simulink model "LugR7sStEnCtrl"  (R2024b)
settings: Solver=FixedStepDiscrete  StartTime=0.0  StopTime=10.0  FixedStep=0.01  RelTol=1e-3
undefined symbols (not defined in the file or in its folder): data, KeSMSw4SSecRwLtStLgrstOtwdInwdClosePos1_Val, KeSMSw4SSecRwLtStLgrstUpwdDnwdClosePos1_Val, KeSMSw4SSecRwLtStLgrstUpwdDnwdClosePos2_Val, SecRwRtStBkReclnEn_Clear, SecRwRtStBkReclnEn_Set, SecRwRtStFwdBkwdEn_Clear, SecRwRtStFwdBkwdEn_Set, SecRwRtStLgrstInwdOtwdEn_Clear, SecRwRtStLgrstInwdOtwdEn_Set, SecRwRtStLgrstUpwdDnwdEn_Clear, SecRwRtStLgrstUpwdDnwdEn_Set, ThdRwRtStBkReclnEn_Clear, ThdRwRtStBkReclnEn_Set, ThdRwRtStCshnFldEn_Clear, ThdRwRtStCshnFldEn_Set, ThdRwRtStFwdBkwdEn_Clear, ThdRwRtStFwdBkwdEn_Set, ZeroREn_Clear, ZeroREn_Set
libraries: simulink x1
settings Model: Creator=sn2xws  LastModifiedBy=sn55gm
settings Model: ModifiedHistory=|
  | 2024.6.19 V1.0.0 模式流程V1.6
  | 2024.8.2 V3.0.0 模式流程V2.0
  | 2024.8.14 V3.0.1 修复三排前后可能不到位置的问题修复
  | 2024.8.16 V3.0.2腿托和腿托延伸的pos1标定连接错误问题修复
  | 2024.8.23 V3.0.3三右靠背折叠后，未调用前后位置的问题修复
  | 2024.8.26 V3.0.4 模式流程V2.4
  | 2024.9.3 V3.0.5 lug 如果三排折叠已到位，第一阶段会动三排往前的问题
  | 2024.11.15 V3.0.6 md8 md9 同时调用导致2R状态到位被清零，三排前后会重试的问题修复
settings SolverCC: AlgebraicLoopSolver=TrustRegion
settings DataIOCC: SaveFormat=StructureWithTime  ReturnWorkspaceOutputs=off
settings OptimizationCC: DefaultParameterBehavior=Inlined  EnhancedBackFolding=on  PassReuseOutputArgsAs=Individual arguments  ZeroExternalMemoryAtStartup=off  ZeroInternalMemoryAtStartup=off  OptimizeBlockOrder=speed  DifferentSizesBufferReuse=on  OptimizationCustomize=off  EfficientTunableParamExpr=on
settings DebuggingCC: ParameterTunabilityLossMsg=error  UnconnectedInputMsg=warning  UnconnectedOutputMsg=warning  UnconnectedLineMsg=warning  ArithmeticOperatorsInVariantConditions=warning
settings ModelReferenceCC: EnableRefExpFcnMdlSchedulingChecks=on
settings SFSimCC: MATLABDynamicMemAlloc=off  CustomCodeUndefinedFunction=UseInterfaceOnly
settings RTWCC: Description=AUTOSAR  SystemTargetFile=autosar.tlc  GenCodeOnly=on  TemplateMakefile=ert_default_tmf  GenerateReport=on  IncludeHyperlinkInReport=on  LaunchReport=on  DataTypeReplacement=CDataTypesFixedWidth  GenerateTraceInfo=on  GenerateTraceReport=on  GenerateTraceReportSl=on  GenerateTraceReportSf=on  GenerateTraceReportEml=on  GPUComputeCapability=3.5
settings CodeAppCC: ForceParamTrailComments=on  IgnoreCustomStorageClasses=off  OperatorAnnotations=on  SimulinkDataObjDesc=on  SFDataObjDesc=on  InsertBlockDesc=on
settings STFCustomTargetCC: TargetLangStandard=C99 (ISO)  MultiwordLength=256  ParMdlRefBuildCompliant=on  CompOptLevelCompliant=on  IncludeMdlTerminateFcn=off  CombineOutputUpdateFcns=on  SuppressErrorStatus=on  ERTCustomFileBanners=on  SupportNonFinite=off  SupportComplex=off  SupportContinuousTime=off  SupportNonInlinedSFcns=off  RemoveResetFunc=on  MATLABClassNameForMDSCustomization=Simulink.SoftwareTarget.ERTCustomization  AutosarCompliant=on  UseToolchainInfoCompliant=on  LookupTableObjectStructAxisOrder=2,1,3,4,...  LUTObjectStructOrderEvenSpacing=Size,Table,Breakpoints  SystemTargetFile=autosar.tlc
settings ERTTargetCC: TargetLangStandard=C99 (ISO)  ConcurrentExecutionCompliant=off  IncludeMdlTerminateFcn=off  SuppressErrorStatus=on  SupportNonFinite=off  SupportComplex=off  ModelStepFunctionPrototypeControlCompliant=off  CPPClassGenCompliant=off  AutosarCompliant=on  LookupTableObjectStructAxisOrder=2,1,3,4,...  LUTObjectStructOrderEvenSpacing=Size,Table,Breakpoints  ERTCustomFileTemplate=example_file_process.tlc  ERTFilePackagingFormat=Compact  BooleanTrueId=TRUE  BooleanFalseId=FALSE  DynamicArrayContainerType=coder::array

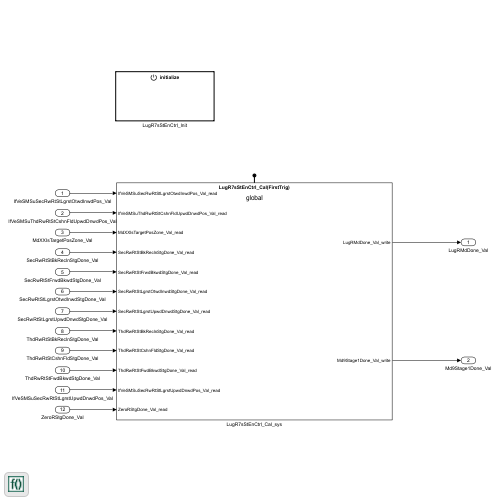
[thumbnail: Simulink's stored preview of the top-level diagram]
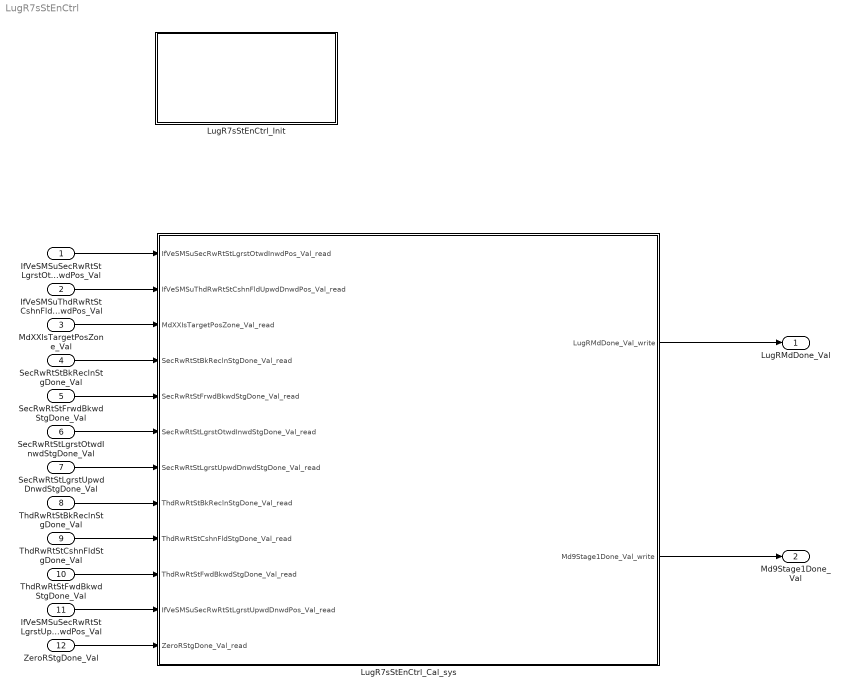
== system LugR7sStEnCtrl ==
  IfVeSMSuSecRwRtStLgrstOtwdInwdPos_Val : Inport  OutDataTypeStr=uint16  PortDimensions=1
  IfVeSMSuThdRwRtStCshnFldUpwdDnwdPos_Val : Inport  Port=2  OutDataTypeStr=uint16  PortDimensions=1
  MdXXIsTargetPosZone_Val : Inport  Port=3  OutDataTypeStr=uint32  PortDimensions=1
  SecRwRtStBkReclnStgDone_Val : Inport  Port=4  OutDataTypeStr=boolean  PortDimensions=1
  SecRwRtStFrwdBkwdStgDone_Val : Inport  Port=5  OutDataTypeStr=boolean  PortDimensions=1
  SecRwRtStLgrstOtwdInwdStgDone_Val : Inport  Port=6  OutDataTypeStr=boolean  PortDimensions=1
  SecRwRtStLgrstUpwdDnwdStgDone_Val : Inport  Port=7  OutDataTypeStr=boolean  PortDimensions=1
  ThdRwRtStBkReclnStgDone_Val : Inport  Port=8  OutDataTypeStr=boolean  PortDimensions=1
  ThdRwRtStCshnFldStgDone_Val : Inport  Port=9  OutDataTypeStr=boolean  PortDimensions=1
  ThdRwRtStFwdBkwdStgDone_Val : Inport  Port=10  OutDataTypeStr=boolean  PortDimensions=1
  IfVeSMSuSecRwRtStLgrstUpwdDnwdPos_Val : Inport  Port=11  OutDataTypeStr=uint16  PortDimensions=1
  ZeroRStgDone_Val : Inport  Port=12  OutDataTypeStr=boolean  PortDimensions=1
  LugR7sStEnCtrl_Cal_sys : Subsystem
  LugR7sStEnCtrl_Init : Subsystem
  LugRMdDone_Val : Outport  OutDataTypeStr=uint8  PortDimensions=1  VectorParamsAs1DForOutWhenUnconnected=off
  Md9Stage1Done_Val : Outport  Port=2  OutDataTypeStr=boolean  PortDimensions=1  VectorParamsAs1DForOutWhenUnconnected=off
  wires:
  IfVeSMSuSecRwRtStLgrstOtwdInwdPos_Val/1 -> LugR7sStEnCtrl_Cal_sys/1(IfVeSMSuSecRwRtStLgrstOtwdInwdPos_Val_read)
  IfVeSMSuThdRwRtStCshnFldUpwdDnwdPos_Val/1 -> LugR7sStEnCtrl_Cal_sys/2(IfVeSMSuThdRwRtStCshnFldUpwdDnwdPos_Val_read)
  MdXXIsTargetPosZone_Val/1 -> LugR7sStEnCtrl_Cal_sys/3(MdXXIsTargetPosZone_Val_read)
  SecRwRtStBkReclnStgDone_Val/1 -> LugR7sStEnCtrl_Cal_sys/4(SecRwRtStBkReclnStgDone_Val_read)
  SecRwRtStFrwdBkwdStgDone_Val/1 -> LugR7sStEnCtrl_Cal_sys/5(SecRwRtStFrwdBkwdStgDone_Val_read)
  SecRwRtStLgrstOtwdInwdStgDone_Val/1 -> LugR7sStEnCtrl_Cal_sys/6(SecRwRtStLgrstOtwdInwdStgDone_Val_read)
  SecRwRtStLgrstUpwdDnwdStgDone_Val/1 -> LugR7sStEnCtrl_Cal_sys/7(SecRwRtStLgrstUpwdDnwdStgDone_Val_read)
  ThdRwRtStBkReclnStgDone_Val/1 -> LugR7sStEnCtrl_Cal_sys/8(ThdRwRtStBkReclnStgDone_Val_read)
  ThdRwRtStCshnFldStgDone_Val/1 -> LugR7sStEnCtrl_Cal_sys/9(ThdRwRtStCshnFldStgDone_Val_read)
  ThdRwRtStFwdBkwdStgDone_Val/1 -> LugR7sStEnCtrl_Cal_sys/10(ThdRwRtStFwdBkwdStgDone_Val_read)
  LugR7sStEnCtrl_Cal_sys/1(LugRMdDone_Val_write) -> LugRMdDone_Val/1
  IfVeSMSuSecRwRtStLgrstUpwdDnwdPos_Val/1 -> LugR7sStEnCtrl_Cal_sys/11(IfVeSMSuSecRwRtStLgrstUpwdDnwdPos_Val_read)
  ZeroRStgDone_Val/1 -> LugR7sStEnCtrl_Cal_sys/12(ZeroRStgDone_Val_read)
  LugR7sStEnCtrl_Cal_sys/2(Md9Stage1Done_Val_write) -> Md9Stage1Done_Val/1

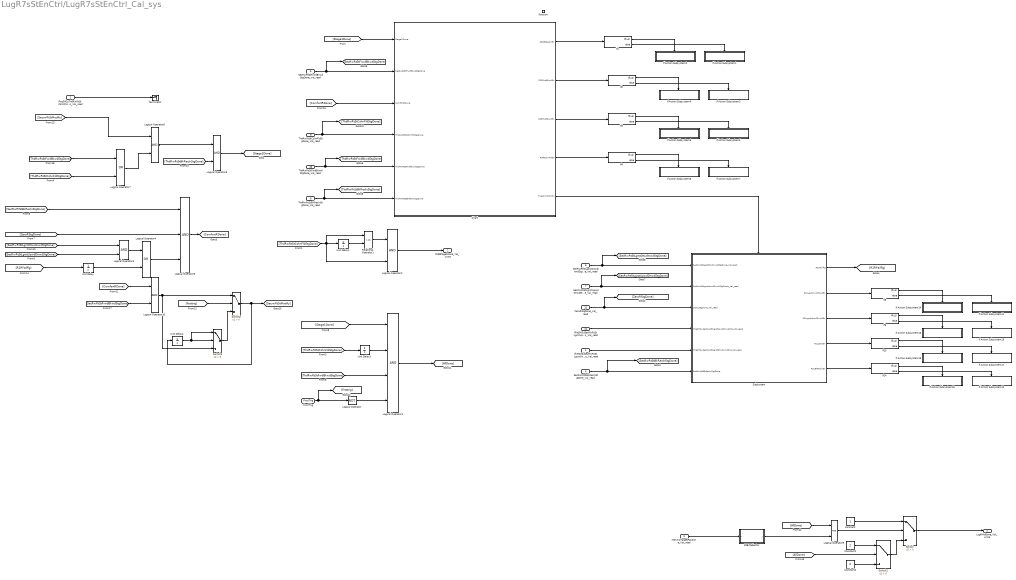
== system LugR7sStEnCtrl/LugR7sStEnCtrl_Cal_sys ==
  IfVeSMSuSecRwRtStLgrstOtwdInwdPos_Val_read : Inport
  IfVeSMSuThdRwRtStCshnFldUpwdDnwdPos_Val_read : Inport  Port=2
  MdXXIsTargetPosZone_Val_read : Inport  Port=3
  SecRwRtStBkReclnStgDone_Val_read : Inport  Port=4
  SecRwRtStFrwdBkwdStgDone_Val_read : Inport  Port=5
  SecRwRtStLgrstOtwdInwdStgDone_Val_read : Inport  Port=6
  SecRwRtStLgrstUpwdDnwdStgDone_Val_read : Inport  Port=7
  ThdRwRtStBkReclnStgDone_Val_read : Inport  Port=8
  ThdRwRtStCshnFldStgDone_Val_read : Inport  Port=9
  ThdRwRtStFwdBkwdStgDone_Val_read : Inport  Port=10
  IfVeSMSuSecRwRtStLgrstUpwdDnwdPos_Val_read : Inport  Port=11
  ZeroRStgDone_Val_read : Inport  Port=12
  function : TriggerPort  TriggerType=function-call  IsSimulinkFunction=on  FunctionName=LugR7sStEnCtrl_Cal  VariantControl=(inherit)
  32BitSelector : Subsystem  mask(32 Bit Selector){BitNum=8}
      mask prompts: BitNum "Select Bit Number"
      mask help: Allows selection of a particular bit (0-31) out of a packed word up to 32 bits long. Output will be true if the bit number selected via the mask parameter is equal to one.
      mask TypeOptions BitNum: 0 | 1 | 2 | 3 | 4 | 5 | 6 | 7 | 8 | 9 | 10 | 11 | 12 | 13 | 14 | 15 | 16 | 17 | 18 | 19 | 20 | 21 | 22 | 23 | 24 | 25 | 26 | 27 | 28 | 29 | 30 | 31
      mask Display:
      | text(0.5, 0.8,'BIT','horizontalAlignment','center')
      | text(0.5, 0.5,'SELECTOR','horizontalAlignment','center')
      | text(0.5, 0.2,['-- Bit ',char(get_param(gcb,'BitNum')),' --'],'horizontalAlignment','center')
  Chart : Stateflow chart  TreatAsAtomicUnit=on
  Constant : Constant  OutDataTypeStr=uint8
  Constant1 : Constant  Value=2  OutDataTypeStr=uint8
  Constant2 : Constant  Value=0  OutDataTypeStr=uint8
  If Action Subsystem1 : Subsystem  TreatAsAtomicUnit=on
  If Action Subsystem11 : Subsystem  TreatAsAtomicUnit=on
  If Action Subsystem12 : Subsystem  TreatAsAtomicUnit=on
  If Action Subsystem14 : Subsystem  TreatAsAtomicUnit=on
  If Action Subsystem15 : Subsystem  TreatAsAtomicUnit=on
  If Action Subsystem16 : Subsystem  TreatAsAtomicUnit=on
  If Action Subsystem17 : Subsystem  TreatAsAtomicUnit=on
  If Action Subsystem18 : Subsystem  TreatAsAtomicUnit=on
  If Action Subsystem2 : Subsystem  TreatAsAtomicUnit=on
  If Action Subsystem25 : Subsystem  TreatAsAtomicUnit=on
  If Action Subsystem3 : Subsystem  TreatAsAtomicUnit=on
  If Action Subsystem4 : Subsystem  TreatAsAtomicUnit=on
  If Action Subsystem5 : Subsystem  TreatAsAtomicUnit=on
  If Action Subsystem6 : Subsystem  TreatAsAtomicUnit=on
  If Action Subsystem7 : Subsystem  TreatAsAtomicUnit=on
  If Action Subsystem8 : Subsystem  TreatAsAtomicUnit=on
  If{1..4,8..10,14} (8 alike) : If  IfExpression=u1
  Logical Operator : Logic  Operator=NOT  AllPortsSameDT=off  OutDataTypeStr=boolean
  Logical Operator1 : Logic  Inputs=4  AllPortsSameDT=off  OutDataTypeStr=boolean
  Logical Operator{2..3,6,8..10} (6 alike) : Logic  AllPortsSameDT=off  OutDataTypeStr=boolean
  Logical Operator4 : Logic  Operator=OR  AllPortsSameDT=off  OutDataTypeStr=boolean
  Logical Operator5 : Logic  Inputs=3  AllPortsSameDT=off  OutDataTypeStr=boolean
  Logical Operator7 : Logic  Operator=OR  AllPortsSameDT=off  OutDataTypeStr=boolean
  Relational Operator1 : RelationalOperator  Operator=~=  OutDataTypeStr=boolean  RndMeth=Simplest  InputSameDT=off
  Subsystem : Subsystem
  Switch{,1..3} (4 alike) : Switch  Criteria=u2 > Threshold  SaturateOnIntegerOverflow=off  InputSameDT=off
  Terminator : Terminator
  Unit Delay{,1..3} (4 alike) : UnitDelay  SampleTime=-1  HasFrameUpgradeWarning=on
  FirstTrig : ArgIn  OutDataTypeStr=boolean  ArgumentName=FirstTrig
  LugRMdDone_Val_write : Outport  VectorParamsAs1DForOutWhenUnconnected=off
      settings: EnsureOutportIsVirtual=on
  Md9Stage1Done_Val_write : Outport  Port=2  VectorParamsAs1DForOutWhenUnconnected=off
      settings: EnsureOutportIsVirtual=on
  wires:
  SecRwRtStBkReclnStgDone_Val_read/1 -> [SecRwRtStBkReclnStgDone], Subsystem/6(SecRwLtStBkReclnStgDone)
  ThdRwRtStCshnFldStgDone_Val_read/1 -> [ThdRwRtStCshnFldStgDone], Chart/4(ThdRwRtStCshnFldStgDone)
  ThdRwRtStFwdBkwdStgDone_Val_read/1 -> [ThdRwRtStFwdBkwdStgDone], Chart/5(ThdRwRtStFwdBkwdStgDone)
  Chart/5(TrigComfortMd()) -> Subsystem/Trigger
  If8/2 -> If Action Subsystem11/Action
  SecRwRtStLgrstOtwdInwdStgDone_Val_read/1 -> [SecRwRtStLgrstOtwdInwdStgDone], Subsystem/1(SecRwLtStLgrstOtwdInwdStgDone_Val_read)
  If14/2 -> If Action Subsystem12/Action
  IfVeSMSuSecRwRtStLgrstOtwdInwdPos_Val_read/1 -> Subsystem/5(IfVeSMSuSecRwLtStLgrstOtwdInwdPos_Val_read)
  Subsystem/3(R2LLgrstUpwdDnwdEn) -> If9/1
  If9/1 -> If Action Subsystem16/Action
  If8/1 -> If Action Subsystem14/Action
  Subsystem/5(R2LBkReclnEn) -> If14/1
  If14/1 -> If Action Subsystem25/Action
  Subsystem/4(R2LZeroEn) -> If10/1
  If10/2 -> If Action Subsystem17/Action
  If9/2 -> If Action Subsystem15/Action
  Subsystem/2(R2LLgrstInwdOtwdEn) -> If8/1
  If10/1 -> If Action Subsystem18/Action
  SecRwRtStLgrstUpwdDnwdStgDone_Val_read/1 -> [SecRwRtStLgrstUpwdDnwdStgDone], Subsystem/2(SecRwLtStLgrstUpwdDnwdStgDone_Val_read)
  Subsystem/1(R2LFailflg) -> [R2RFailflg]
  IfVeSMSuSecRwRtStLgrstUpwdDnwdPos_Val_read/1 -> Subsystem/4(IfVeSMSuSecRwLtStLgrstUpwdDnwdPos_Val_read)
  SecRwRtStFrwdBkwdStgDone_Val_read/1 -> [SecRwRtStFrwdBkwdStgDone], Chart/2(SecRwRtStFrwdBkwdStgDone)
  ThdRwRtStBkReclnStgDone_Val_read/1 -> [ThdRwRtStBkReclnStgDone], Chart/6(ThdRwRtStBkReclnStgDone)
  Logical Operator8/1 -> Logical Operator6/1
  IfVeSMSuThdRwRtStCshnFldUpwdDnwdPos_Val_read/1 -> Terminator/1
  [Stage1Done] -> Chart/1(Stage1Done)
  Unit Delay/1 -> Logical Operator4/2
  Logical Operator5/1 -> [ComfortRDone]
  [SecRwRtStBkReclnStgDone] -> Logical Operator5/1
  [SecRwRtStLgrstUpwdDnwdStgDone] -> Logical Operator3/2
  [R2RFailflg] -> Unit Delay/1
  [ZeroRStgDone] -> Logical Operator5/2
  [SecRwRtStLgrstOtwdInwdStgDone] -> Logical Operator3/1
  Logical Operator4/1 -> Logical Operator5/3
  Logical Operator3/1 -> Logical Operator4/1
  [ComfortRDone] -> Chart/3(ComfortRDone)
  Constant1/1 -> Switch1/1
  MdXXIsTargetPosZone_Val_read/1 -> 32BitSelector/1(x)
  32BitSelector/1(y) -> Logical Operator9/2
  Logical Operator9/1 -> Switch/2
  Switch1/1 -> Switch/3
  Constant2/1 -> Switch1/3
  Switch/1 -> LugRMdDone_Val_write/1
  Constant/1 -> Switch/1
  [AllDone] -> Switch1/2
  [AllDone] -> Logical Operator9/1
  Logical Operator1/1 -> [AllDone]
  [Stage1Done] -> Logical Operator1/1
  ZeroRStgDone_Val_read/1 -> [ZeroRStgDone], Subsystem/3(ZeroLStgDone_Val_read)
  If1/1 -> If Action Subsystem2/Action
  If1/2 -> If Action Subsystem1/Action
  Chart/1(R3RBkReclnEn) -> If1/1
  Chart/2(R2RFwdBkwdEn) -> If2/1
  If2/2 -> If Action Subsystem3/Action
  If2/1 -> If Action Subsystem4/Action
  If3/1 -> If Action Subsystem6/Action
  If3/2 -> If Action Subsystem5/Action
  Chart/3(R3RFwdBkwdEn) -> If3/1
  Chart/4(R3RCshnFldEn) -> If4/1
  If4/2 -> If Action Subsystem7/Action
  If4/1 -> If Action Subsystem8/Action
  Unit Delay1/1 -> Relational Operator1/2
  Logical Operator2/1 -> Md9Stage1Done_Val_write/1
  Relational Operator1/1 -> Logical Operator2/1
  [ThdRwRtStCshnFldStgDone] -> Relational Operator1/1, Logical Operator2/2, Unit Delay1/1
  Logical Operator6/1 -> [Stage1Done]
  [ThdRwRtStBkReclnStgDone] -> Logical Operator6/2
  Unit Delay3/1 -> Logical Operator1/2
  FirstTrig/1 -> [firsttrig], Logical Operator/1
  Logical Operator/1 -> Logical Operator1/4
  Logical Operator7/1 -> Logical Operator8/2
  [ThdRwRtStFwdBkwdStgDone] -> Logical Operator7/1
  [ThdRwRtStCshnFldStgDone] -> Logical Operator7/2
  [ThdRwRtStCshnFldStgDone] -> Unit Delay3/1
  [ThdRwRtStFwdBkwdStgDone] -> Logical Operator1/3
  [firsttrig] -> Switch2/2
  Unit Delay2/1 -> Switch3/1, Switch3/2
  Switch2/1 -> Unit Delay2/1, [SecrwRtStModify]
  Logical Operator10/1 -> Switch3/3, Switch2/1
  Switch3/1 -> Switch2/3
  [ComfortRDone] -> Logical Operator10/1
  [SecRwRtStFrwdBkwdStgDone] -> Logical Operator10/2
  [SecrwRtStModify] -> Logical Operator8/1

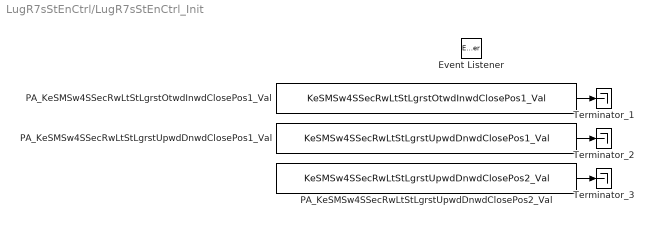
== system LugR7sStEnCtrl/LugR7sStEnCtrl_Init ==
  Event Listener : EventListener  EventName=reset
  PA_KeSMSw4SSecRwLtStLgrstOtwdInwdClosePos1_Val : Constant  Value=KeSMSw4SSecRwLtStLgrstOtwdInwdClosePos1_Val
  PA_KeSMSw4SSecRwLtStLgrstUpwdDnwdClosePos1_Val : Constant  Value=KeSMSw4SSecRwLtStLgrstUpwdDnwdClosePos1_Val
  PA_KeSMSw4SSecRwLtStLgrstUpwdDnwdClosePos2_Val : Constant  Value=KeSMSw4SSecRwLtStLgrstUpwdDnwdClosePos2_Val
  Terminator_1 : Terminator
  Terminator_2 : Terminator
  Terminator_3 : Terminator
  wires:
  PA_KeSMSw4SSecRwLtStLgrstOtwdInwdClosePos1_Val/1 -> Terminator_1/1
  PA_KeSMSw4SSecRwLtStLgrstUpwdDnwdClosePos1_Val/1 -> Terminator_2/1
  PA_KeSMSw4SSecRwLtStLgrstUpwdDnwdClosePos2_Val/1 -> Terminator_3/1

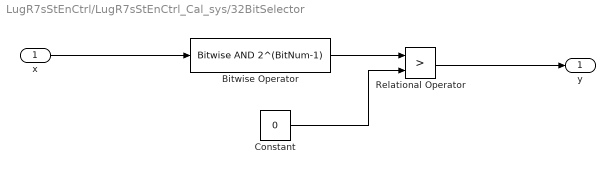
== system LugR7sStEnCtrl/LugR7sStEnCtrl_Cal_sys/32BitSelector ==
  x : Inport
  Bitwise Operator : simulink/Logic and Bit Operations/Bitwise Operator  logicop=AND  UseBitMask=on  BitMask=2^(BitNum-1)  BitMaskRealWorld=Stored Integer
  Constant : Constant  Value=0  OutDataTypeStr=uint32
  Relational Operator : RelationalOperator  Operator=>  OutDataTypeStr=boolean  RndMeth=Simplest  InputSameDT=off
  y : Outport  VectorParamsAs1DForOutWhenUnconnected=off
  wires:
  Relational Operator/1 -> y/1
  Constant/1 -> Relational Operator/2
  x/1 -> Bitwise Operator/1
  Bitwise Operator/1 -> Relational Operator/1

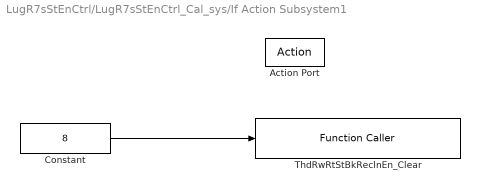
== system LugR7sStEnCtrl/LugR7sStEnCtrl_Cal_sys/If Action Subsystem1 ==
  Action Port : ActionPort  ActionPortLabel=else
  Constant : Constant  Value=8  OutDataTypeStr=uint8
  ThdRwRtStBkReclnEn_Clear : FunctionCaller  FunctionPrototype=ThdRwRtStBkReclnEn_Clear(data)  InputArgumentSpecifications=uint8(1)  OutputArgumentSpecifications=<Enter example>
  wires:
  Constant/1 -> ThdRwRtStBkReclnEn_Clear/1

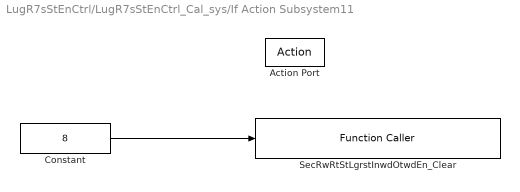
== system LugR7sStEnCtrl/LugR7sStEnCtrl_Cal_sys/If Action Subsystem11 ==
  Action Port : ActionPort  ActionPortLabel=else
  Constant : Constant  Value=8  OutDataTypeStr=uint8
  SecRwRtStLgrstInwdOtwdEn_Clear : FunctionCaller  FunctionPrototype=SecRwRtStLgrstInwdOtwdEn_Clear(data)  InputArgumentSpecifications=uint8(1)  OutputArgumentSpecifications=<Enter example>
  wires:
  Constant/1 -> SecRwRtStLgrstInwdOtwdEn_Clear/1

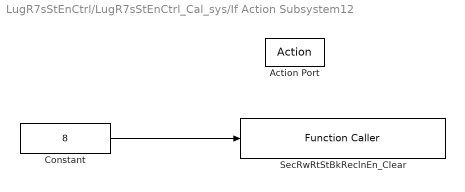
== system LugR7sStEnCtrl/LugR7sStEnCtrl_Cal_sys/If Action Subsystem12 ==
  Action Port : ActionPort  ActionPortLabel=else
  Constant : Constant  Value=8  OutDataTypeStr=uint8
  SecRwRtStBkReclnEn_Clear : FunctionCaller  FunctionPrototype=SecRwRtStBkReclnEn_Clear(data)  InputArgumentSpecifications=uint8(1)  OutputArgumentSpecifications=<Enter example>
  wires:
  Constant/1 -> SecRwRtStBkReclnEn_Clear/1

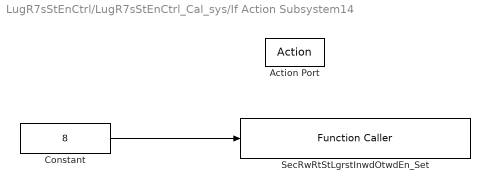
== system LugR7sStEnCtrl/LugR7sStEnCtrl_Cal_sys/If Action Subsystem14 ==
  Action Port : ActionPort  ActionPortLabel=if(u1)
  Constant : Constant  Value=8  OutDataTypeStr=uint8
  SecRwRtStLgrstInwdOtwdEn_Set : FunctionCaller  FunctionPrototype=SecRwRtStLgrstInwdOtwdEn_Set(data)  InputArgumentSpecifications=uint8(1)  OutputArgumentSpecifications=<Enter example>
  wires:
  Constant/1 -> SecRwRtStLgrstInwdOtwdEn_Set/1

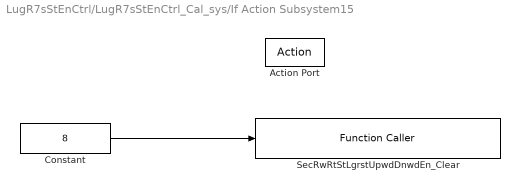
== system LugR7sStEnCtrl/LugR7sStEnCtrl_Cal_sys/If Action Subsystem15 ==
  Action Port : ActionPort  ActionPortLabel=else
  Constant : Constant  Value=8  OutDataTypeStr=uint8
  SecRwRtStLgrstUpwdDnwdEn_Clear : FunctionCaller  FunctionPrototype=SecRwRtStLgrstUpwdDnwdEn_Clear(data)  InputArgumentSpecifications=uint8(1)  OutputArgumentSpecifications=<Enter example>
  wires:
  Constant/1 -> SecRwRtStLgrstUpwdDnwdEn_Clear/1

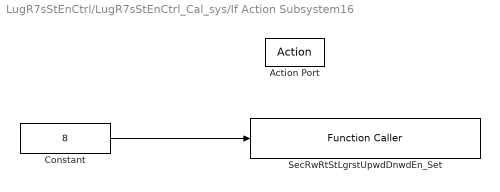
== system LugR7sStEnCtrl/LugR7sStEnCtrl_Cal_sys/If Action Subsystem16 ==
  Action Port : ActionPort  ActionPortLabel=if(u1)
  Constant : Constant  Value=8  OutDataTypeStr=uint8
  SecRwRtStLgrstUpwdDnwdEn_Set : FunctionCaller  FunctionPrototype=SecRwRtStLgrstUpwdDnwdEn_Set(data)  InputArgumentSpecifications=uint8(1)  OutputArgumentSpecifications=<Enter example>
  wires:
  Constant/1 -> SecRwRtStLgrstUpwdDnwdEn_Set/1

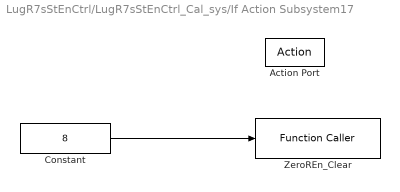
== system LugR7sStEnCtrl/LugR7sStEnCtrl_Cal_sys/If Action Subsystem17 ==
  Action Port : ActionPort  ActionPortLabel=else
  Constant : Constant  Value=8  OutDataTypeStr=uint8
  ZeroREn_Clear : FunctionCaller  FunctionPrototype=ZeroREn_Clear(data)  InputArgumentSpecifications=uint8(1)  OutputArgumentSpecifications=<Enter example>
  wires:
  Constant/1 -> ZeroREn_Clear/1

== system LugR7sStEnCtrl/LugR7sStEnCtrl_Cal_sys/If Action Subsystem18 ==
  Action Port : ActionPort  ActionPortLabel=if(u1)
  Constant : Constant  Value=8  OutDataTypeStr=uint8
  ZeroREn_Set : FunctionCaller  FunctionPrototype=ZeroREn_Set(data)  InputArgumentSpecifications=uint8(1)  OutputArgumentSpecifications=<Enter example>
  wires:
  Constant/1 -> ZeroREn_Set/1

== system LugR7sStEnCtrl/LugR7sStEnCtrl_Cal_sys/If Action Subsystem2 ==
  Action Port : ActionPort  ActionPortLabel=if(u1)
  Constant : Constant  Value=8  OutDataTypeStr=uint8
  ThdRwRtStBkReclnEn_Set : FunctionCaller  FunctionPrototype=ThdRwRtStBkReclnEn_Set(data)  InputArgumentSpecifications=uint8(1)  OutputArgumentSpecifications=<Enter example>
  wires:
  Constant/1 -> ThdRwRtStBkReclnEn_Set/1

== system LugR7sStEnCtrl/LugR7sStEnCtrl_Cal_sys/If Action Subsystem25 ==
  Action Port : ActionPort  ActionPortLabel=if(u1)
  Constant : Constant  Value=8  OutDataTypeStr=uint8
  SecRwRtStBkReclnEn_Set : FunctionCaller  FunctionPrototype=SecRwRtStBkReclnEn_Set(data)  InputArgumentSpecifications=uint8(1)  OutputArgumentSpecifications=<Enter example>
  wires:
  Constant/1 -> SecRwRtStBkReclnEn_Set/1

== system LugR7sStEnCtrl/LugR7sStEnCtrl_Cal_sys/If Action Subsystem3 ==
  Action Port : ActionPort  ActionPortLabel=else
  Constant : Constant  Value=8  OutDataTypeStr=uint8
  SecRwRtStFwdBkwdEn_Clear : FunctionCaller  FunctionPrototype=SecRwRtStFwdBkwdEn_Clear(data)  InputArgumentSpecifications=uint8(1)  OutputArgumentSpecifications=<Enter example>
  wires:
  Constant/1 -> SecRwRtStFwdBkwdEn_Clear/1

== system LugR7sStEnCtrl/LugR7sStEnCtrl_Cal_sys/If Action Subsystem4 ==
  Action Port : ActionPort  ActionPortLabel=if(u1)
  Constant : Constant  Value=8  OutDataTypeStr=uint8
  SecRwRtStFwdBkwdEn_Set : FunctionCaller  FunctionPrototype=SecRwRtStFwdBkwdEn_Set(data)  InputArgumentSpecifications=uint8(1)  OutputArgumentSpecifications=<Enter example>
  wires:
  Constant/1 -> SecRwRtStFwdBkwdEn_Set/1

== system LugR7sStEnCtrl/LugR7sStEnCtrl_Cal_sys/If Action Subsystem5 ==
  Action Port : ActionPort  ActionPortLabel=else
  Constant : Constant  Value=8  OutDataTypeStr=uint8
  ThdRwRtStFwdBkwdEn_Clear : FunctionCaller  FunctionPrototype=ThdRwRtStFwdBkwdEn_Clear(data)  InputArgumentSpecifications=uint8(1)  OutputArgumentSpecifications=<Enter example>
  wires:
  Constant/1 -> ThdRwRtStFwdBkwdEn_Clear/1

== system LugR7sStEnCtrl/LugR7sStEnCtrl_Cal_sys/If Action Subsystem6 ==
  Action Port : ActionPort  ActionPortLabel=if(u1)
  Constant : Constant  Value=8  OutDataTypeStr=uint8
  ThdRwRtStFwdBkwdEn_Set : FunctionCaller  FunctionPrototype=ThdRwRtStFwdBkwdEn_Set(data)  InputArgumentSpecifications=uint8(1)  OutputArgumentSpecifications=<Enter example>
  wires:
  Constant/1 -> ThdRwRtStFwdBkwdEn_Set/1

== system LugR7sStEnCtrl/LugR7sStEnCtrl_Cal_sys/If Action Subsystem7 ==
  Action Port : ActionPort  ActionPortLabel=else
  Constant : Constant  Value=8  OutDataTypeStr=uint8
  ThdRwRtStCshnFldEn_Clear : FunctionCaller  FunctionPrototype=ThdRwRtStCshnFldEn_Clear(data)  InputArgumentSpecifications=uint8(1)  OutputArgumentSpecifications=<Enter example>
  wires:
  Constant/1 -> ThdRwRtStCshnFldEn_Clear/1

== system LugR7sStEnCtrl/LugR7sStEnCtrl_Cal_sys/If Action Subsystem8 ==
  Action Port : ActionPort  ActionPortLabel=if(u1)
  Constant : Constant  Value=8  OutDataTypeStr=uint8
  ThdRwRtStCshnFldEn_Set : FunctionCaller  FunctionPrototype=ThdRwRtStCshnFldEn_Set(data)  InputArgumentSpecifications=uint8(1)  OutputArgumentSpecifications=<Enter example>
  wires:
  Constant/1 -> ThdRwRtStCshnFldEn_Set/1

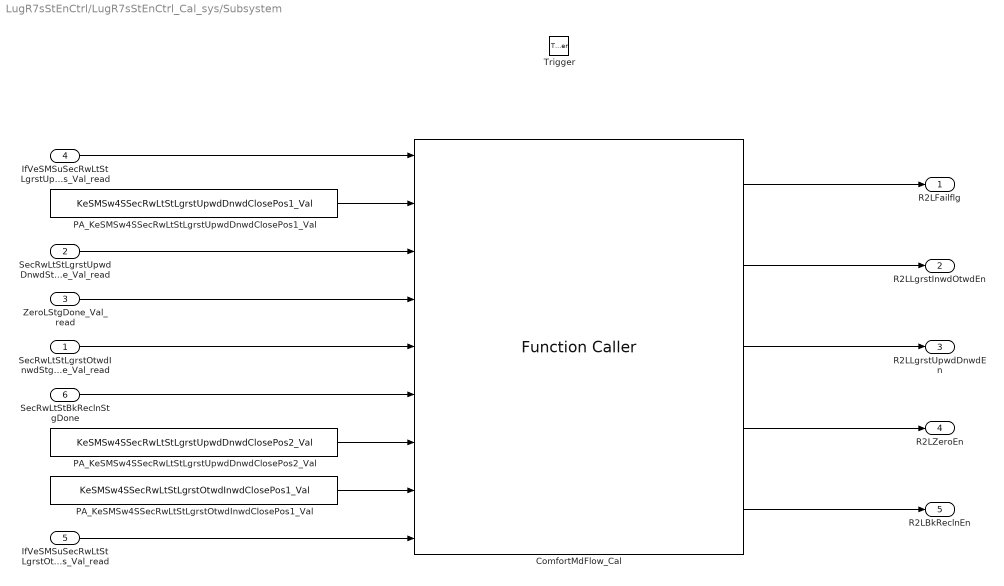
== system LugR7sStEnCtrl/LugR7sStEnCtrl_Cal_sys/Subsystem ==
  SecRwLtStLgrstOtwdInwdStgDone_Val_read : Inport
  SecRwLtStLgrstUpwdDnwdStgDone_Val_read : Inport  Port=2
  ZeroLStgDone_Val_read : Inport  Port=3
  IfVeSMSuSecRwLtStLgrstUpwdDnwdPos_Val_read : Inport  Port=4
  IfVeSMSuSecRwLtStLgrstOtwdInwdPos_Val_read : Inport  Port=5
  SecRwLtStBkReclnStgDone : Inport  Port=6
  Trigger : TriggerPort  TriggerType=function-call  VariantControl=Variant  PortDimensions=1
  ComfortMdFlow_Cal : FunctionCaller  FunctionPrototype=[Failflg,LgrstInwdOtwdEn,LgrstUpwdDnwdEn,ZeroEn,BkReclnEn] = ComfortMdFlow_Cal(LgrstUpwdDnwdPos,LgrstUpwdDnwdClosePos1,LgrstUpwdStgDone,ZeroStgDone,LgrstInwdStgDone,BkReclnStgDone,LgrstUpwdDnwdClosePos2,LgrstInwdOtwdClosePos1,LgrstInwdOtwdPos)  InputArgumentSpecifications=uint16(1), uint16(1), boolean(true), boolean(true), boolean(true), boolean(true), uint16(1), uint16(1), uint16(1)  OutputArgumentSpecifications=boolean(true), boolean(true), boolean(true), boolean(true), boolean(true)
  PA_KeSMSw4SSecRwLtStLgrstOtwdInwdClosePos1_Val : Constant  Value=KeSMSw4SSecRwLtStLgrstOtwdInwdClosePos1_Val
  PA_KeSMSw4SSecRwLtStLgrstUpwdDnwdClosePos1_Val : Constant  Value=KeSMSw4SSecRwLtStLgrstUpwdDnwdClosePos1_Val
  PA_KeSMSw4SSecRwLtStLgrstUpwdDnwdClosePos2_Val : Constant  Value=KeSMSw4SSecRwLtStLgrstUpwdDnwdClosePos2_Val
  R2LFailflg : Outport  VectorParamsAs1DForOutWhenUnconnected=off
  R2LLgrstInwdOtwdEn : Outport  Port=2  VectorParamsAs1DForOutWhenUnconnected=off
  R2LLgrstUpwdDnwdEn : Outport  Port=3  VectorParamsAs1DForOutWhenUnconnected=off
  R2LZeroEn : Outport  Port=4  VectorParamsAs1DForOutWhenUnconnected=off
  R2LBkReclnEn : Outport  Port=5  VectorParamsAs1DForOutWhenUnconnected=off
  wires:
  SecRwLtStBkReclnStgDone/1 -> ComfortMdFlow_Cal/6
  PA_KeSMSw4SSecRwLtStLgrstUpwdDnwdClosePos2_Val/1 -> ComfortMdFlow_Cal/7
  IfVeSMSuSecRwLtStLgrstUpwdDnwdPos_Val_read/1 -> ComfortMdFlow_Cal/1
  SecRwLtStLgrstUpwdDnwdStgDone_Val_read/1 -> ComfortMdFlow_Cal/3
  IfVeSMSuSecRwLtStLgrstOtwdInwdPos_Val_read/1 -> ComfortMdFlow_Cal/9
  SecRwLtStLgrstOtwdInwdStgDone_Val_read/1 -> ComfortMdFlow_Cal/5
  ZeroLStgDone_Val_read/1 -> ComfortMdFlow_Cal/4
  ComfortMdFlow_Cal/2 -> R2LLgrstInwdOtwdEn/1
  ComfortMdFlow_Cal/4 -> R2LZeroEn/1
  ComfortMdFlow_Cal/5 -> R2LBkReclnEn/1
  ComfortMdFlow_Cal/3 -> R2LLgrstUpwdDnwdEn/1
  ComfortMdFlow_Cal/1 -> R2LFailflg/1
  PA_KeSMSw4SSecRwLtStLgrstUpwdDnwdClosePos1_Val/1 -> ComfortMdFlow_Cal/2
  PA_KeSMSw4SSecRwLtStLgrstOtwdInwdClosePos1_Val/1 -> ComfortMdFlow_Cal/8

== stateflow chart LugR7sStEnCtrl/LugR7sStEnCtrl_Cal_sys/Chart ==
  (default) -> (junction 1) : {
      | R3RBkReclnEn =0;
      | R3RCshnFldEn = 0;
      | R3RFwdBkwdEn = 0;
      | R3RFwdBkwdEn =0;
      | R2RFwdBkwdEn = 0;
      | }
  (junction 1) -> (junction 3) [order 1] : [Stage1Done]
  (junction 3) -> (junction 208) [order 1] : [ThdRwRtStCshnFldStgDone]
  (junction 1) -> (junction 216) [order 2] : {
      | TrigComfortMd;
      | }
  (junction 3) -> (junction 7) [order 2] : {
      | R3RCshnFldEn = 1;
      | }
  (junction 208) -> (junction 289)
  (junction 216) -> (junction 235)
  (junction 235) -> (junction 248)
  (junction 248) -> (junction 250) [order 1] : [ComfortRDone]
  (junction 250) -> (junction 254) [order 1] : [SecRwRtStFrwdBkwdStgDone]
  (junction 248) -> (junction 262) [order 2]
  (junction 250) -> (junction 266) [order 2] : {
      | R2RFwdBkwdEn =1;
      | }
  (junction 254) -> (junction 259)
  (junction 266) -> (junction 262)
  (junction 259) -> (junction 266)
  (junction 262) -> (junction 221)
  (junction 221) -> (junction 223) [order 1] : [!ThdRwRtStBkReclnStgDone]
  (junction 221) -> (junction 334) [order 2]
  (junction 223) -> (junction 335) : {R3RBkReclnEn =1;}
  (junction 334) -> (junction 333) [order 1] : [ThdRwRtStFwdBkwdStgDone||ThdRwRtStCshnFldStgDone]
  (junction 334) -> (junction 244) [order 2] : {
      | R3RFwdBkwdEn=1;
      | }
  (junction 333) -> (junction 336)
  (junction 336) -> (junction 244)
  (junction 335) -> (junction 336)
  (junction 7) -> (junction 335)
  (junction 289) -> (junction 7)
  (junction 244) -> (junction 299)
  (junction 299) -> (junction 314) [order 1] : [ThdRwRtStCshnFldStgDone&&Stage1Done]
  (junction 314) -> (junction 344) [order 1] : [(ThdRwRtStFwdBkwdStgDone)]
  (junction 299) -> (junction 318) [order 2]
  (junction 314) -> (junction 320) [order 2] : {
      | R3RFwdBkwdEn=1;
      | }
  (junction 344) -> (junction 346)
  (junction 320) -> (junction 318)
  (junction 346) -> (junction 320)
  data: Stage1Done input boolean; R3RBkReclnEn output boolean; R2RFwdBkwdEn output boolean; SecRwRtStFrwdBkwdStgDone input; ComfortRDone input; R3RFwdBkwdEn output boolean; R3RCshnFldEn output boolean; ThdRwRtStCshnFldStgDone input; ThdRwRtStFwdBkwdStgDone input; ThdRwRtStBkReclnStgDone input
  events: TrigComfortMd output FUNCTION_CALL_EVENT
